simulink subsystem "SchlittenGleichungKraft"  (R2020a)
settings: Solver=VariableStepAuto  StartTime=0.0  StopTime=10.0  RelTol=1e-3
settings Model: Creator=Tobias  LastModifiedBy=Tobias

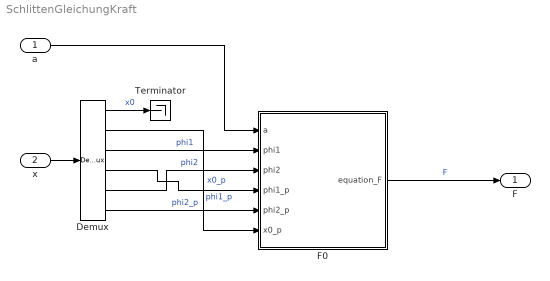
== system SchlittenGleichungKraft ==
  a : Inport
  x : Inport  Port=2
  Demux : Demux  Outputs=6
  F0 : MATLAB Function  TreatAsAtomicUnit=on
  Terminator : Terminator
  F : Outport
  wires:
  Demux/5 -> F0/3(phi2)  "phi2"
  F0/1(equation_F) -> F/1  "F"
  a/1 -> F0/1(a)
  Demux/1 -> Terminator/1  "x0"
  Demux/2 -> F0/6(x0_p)  "x0_p"
  Demux/4 -> F0/4(phi1_p)  "phi1_p"
  x/1 -> Demux/1
  Demux/6 -> F0/5(phi2_p)  "phi2_p"
  Demux/3 -> F0/2(phi1)  "phi1"

== matlab function SchlittenGleichungKraft/F0 ==
  data: a input; equation_F output; phi1 input; phi2 input; phi1_p input; phi2_p input; x0_p input
function equation_F = F0(a,phi1,phi2,phi1_p,phi2_p,x0_p)
%#codegen

%    This function was generated by the Symbolic Math Toolbox version 8.5.
%    29-Sep-2020 14:39:34

t2 = cos(phi1);
t3 = cos(phi2);
t4 = phi1.*2.0;
t5 = phi2.*2.0;
t6 = phi1_p.^2;
t7 = phi2_p.^2;
t10 = -phi2;
t12 = x0_p.*1.0e+2;
t8 = cos(t4);
t9 = cos(t5);
t11 = -t5;
t13 = tanh(t12);
t16 = t4+t10;
t14 = phi1+t11;
t17 = t4+t11;
t18 = cos(t16);
t20 = t9.*7.725321288105266e-6;
t21 = t8.*2.018491701133292e-4;
t15 = cos(t14);
t19 = cos(t17);
t22 = -t20;
t23 = t19.*2.774599575275721e-3;
t24 = t21+t22+t23-1.198618363017405e-2;
equation_F = (t24.*(a-(t13.*9.299881906349582e-3+x0_p.*1.177200241310074e-2-sin(t4).*1.98014035881176e-3+sin(t5).*7.578540183631266e-5+phi1_p.*t2.*2.137521421079153e-5-phi1_p.*t3.*5.98704681211936e-7-phi2_p.*t2.*7.648381732674934e-7+phi2_p.*t3.*5.98704681211936e-7-phi1_p.*t15.*4.591026674209762e-6+phi2_p.*t15.*1.642740241242664e-7+phi1_p.*t18.*6.961035565679671e-7-phi2_p.*t18.*6.961035565679671e-7-t13.*t19.*2.182976984578489e-3-t19.*x0_p.*2.763262005795555e-3+t6.*sin(phi1).*1.036999344477642e-4+t7.*sin(phi2).*1.052517194912801e-5+t6.*sin(t14).*2.178540603245685e-6+t7.*sin(t16).*1.343294138643462e-5)./t24))./(t19.*1.625448238703268e-4-6.924707301823963e-4);
